simulink model "VoltageRegulator"  (R2018a)
settings: Solver=VariableStepAuto  StartTime=0.0  StopTime=10.0  RelTol=1e-3
libraries: elec_lib x6, pe_lib x4, fl_lib x3, nesl_utility x3
settings Model: Creator=Jayef  LastModifiedBy=Jayef

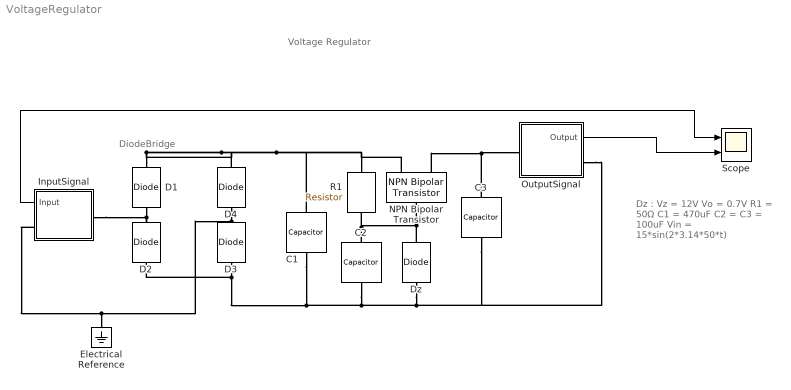
== system VoltageRegulator ==
  note: Voltage Regulator
  note: DiodeBridge
  note: Dz :
      | Vz = 12V
      | Vo = 0.7V
      |
      | R1 = 50Ω C1 = 470uF
      |
      | C2 = C3 = 100uF
      |
      | Vin = 15*sin(2*3.14*50*t)
  C1 : elec_lib/Passive Devices/Capacitor  enable_table=0  c=470 uF  Cvec=[1e-05, 1e-06] F  Vvec=[0, 10] V  CV_table_symmetry=1  C_tol=5  enable_C_tol=0  tol_distribution=1  nSigma=4  r=1e-6 Ohm  g=0 1/Ohm  enable_operating_limits=0  operating_limit_action=2  max_working_voltage_range=[-25, 25] V  power_rating=1 W  enable_faults=0  fault_action=1  Cscale_faulted=100  R_faulted=1e-3 Ohm  G_faulted=0 1/Ohm  tau_fault=1e-3 s  enable_temporal_fault=0  t_fault=1 s  enable_behavioral_fault=0  max_permissible_voltage_range=[-100, 100] V  t_fail_on_voltage=1 s  i_specify=off  i_priority=None  i=0 A  i_nominal_specify=off  i_nominal_unit=A  i_nominal_value=1  v_specify=off  v_priority=None  v=0 V  v_nominal_specify=off  v_nominal_unit=V  v_nominal_value=1  vc_specify=off  vc_priority=High  vc=0 V  vc_nominal_specify=off  vc_nominal_unit=V  vc_nominal_value=1
  C2 : elec_lib/Passive Devices/Capacitor  enable_table=0  c=100 uF  Cvec=[1e-05, 1e-06] F  Vvec=[0, 10] V  CV_table_symmetry=1  C_tol=5  enable_C_tol=0  tol_distribution=1  nSigma=4  r=1e-6 Ohm  g=0 1/Ohm  enable_operating_limits=0  operating_limit_action=2  max_working_voltage_range=[-25, 25] V  power_rating=1 W  enable_faults=0  fault_action=1  Cscale_faulted=100  R_faulted=1e-3 Ohm  G_faulted=0 1/Ohm  tau_fault=1e-3 s  enable_temporal_fault=0  t_fault=1 s  enable_behavioral_fault=0  max_permissible_voltage_range=[-100, 100] V  t_fail_on_voltage=1 s  i_specify=off  i_priority=None  i=0 A  i_nominal_specify=off  i_nominal_unit=A  i_nominal_value=1  v_specify=off  v_priority=None  v=0 V  v_nominal_specify=off  v_nominal_unit=V  v_nominal_value=1  vc_specify=off  vc_priority=High  vc=0 V  vc_nominal_specify=off  vc_nominal_unit=V  vc_nominal_value=1
  C3 : elec_lib/Passive Devices/Capacitor  enable_table=0  c=100 uF  Cvec=[1e-05, 1e-06] F  Vvec=[0, 10] V  CV_table_symmetry=1  C_tol=5  enable_C_tol=0  tol_distribution=1  nSigma=4  r=1e-6 Ohm  g=0 1/Ohm  enable_operating_limits=0  operating_limit_action=2  max_working_voltage_range=[-25, 25] V  power_rating=1 W  enable_faults=0  fault_action=1  Cscale_faulted=100  R_faulted=1e-3 Ohm  G_faulted=0 1/Ohm  tau_fault=1e-3 s  enable_temporal_fault=0  t_fault=1 s  enable_behavioral_fault=0  max_permissible_voltage_range=[-100, 100] V  t_fail_on_voltage=1 s  i_specify=off  i_priority=None  i=0 A  i_nominal_specify=off  i_nominal_unit=A  i_nominal_value=1  v_specify=off  v_priority=None  v=0 V  v_nominal_specify=off  v_nominal_unit=V  v_nominal_value=1  vc_specify=off  vc_priority=High  vc=0 V  vc_nominal_specify=off  vc_nominal_unit=V  vc_nominal_value=1
  D{1..4} (4 alike) : pe_lib/Semiconductors/Fundamental Components/Diode  Vf=0.7 V  Ron=0.3 Ohm  Goff=1e-5 1/Ohm  N_series=1  N_parallel=1  Vf_equiv=0.8 V  Ron_equiv=0.001 Ohm  Goff_equiv=1e-5 1/Ohm
      settings: SourceProductName=Simscape Power Systems  SourceProductBaseCode=PS
  Dz : elec_lib/Semiconductor Devices/Diode  ModelType=2  Vf=.7 V  Ron=0.3 Ohm  Goff=1e-8 S  Rz=0.3 Ohm  Vz=12 V  C_PWL=5 pF  prmExp=1  I12=[.0137, .545] A  V12=[.6, .7] V  I1=0.0137 A  V1=0.6 V  IS=1e-12 A  ec=1  RS=0.01 Ohm  Tmeas=25 degC  BV=inf V  C_param=1  CJ0=5 pF  VJ=1 V  Mgrad=0.5  Vvec=[.1, 10, 100] V  Cvec=[3.5, 1, .4] pF  FC=0.5  Q_param=1  Irrm=-7.15 A  iF=4 A  didt=-750 A/us  trr=115 ns  TT=50 ns  tau=100 ns  T_param=1  IS_T2=1.25e-7 A  I1_T2=0.245 A  V1_T2=0.5 V  Tmeas2=125 degC  EG_param=1  EG=1.11 eV  XTI_param=1  XTI=3  dBVdT=0 V/K  Tdevice=25 degC  i_capacitor_specify=off  i_capacitor_priority=High  i_capacitor=0 A  i_capacitor_nominal_specify=off  i_capacitor_nominal_unit=A  i_capacitor_nominal_value=1  v_capacitor_specify=off  v_capacitor_priority=None  v_capacitor=0 V  v_capacitor_nominal_specify=off  v_capacitor_nominal_unit=V  v_capacitor_nominal_value=1  Rth=[0, 10] K/W  thermal_mass_parameterization=1  thermal_mass=[0, 1] J/K  thermal_time_constant=[0, 10] s  thermal_mass_initial_temperatures=[25, 25] degC
      settings: SourceProductName=Simscape Electronics  SourceProductBaseCode=SN
  Electrical Reference : fl_lib/Electrical/Electrical Elements/Electrical Reference
  InputSignal : Subsystem
  NPN Bipolar Transistor : elec_lib/Semiconductor Devices/NPN Bipolar Transistor  parameterization=1  prmDatasheet=1  prmEquCoeff=1  BF=100  IS=1e-14 A  ec=1  VAF=200 V  hfe=100  hoe=5e-5 1/Ohm  Ic_h=1 mA  Vce_h=5 V  V1=0.55 V  I1=0.5 mA  BR=1  Tmeas=25 degC  RC=0.01 Ohm  RE=1e-4 Ohm  RB=1 Ohm  C_BC=5 pF  C_BE=5 pF  TF=0 us  TR=0 us  hfe_T2=125  XTB=0  V1_T2=0.45 V  I1_T2=0.5 mA  Tmeas2=125 degC  EG=1.11 eV  XTI=3  TdeviceDatasheet=25 degC  TdeviceEquCoeff=25 degC  Rth=[ 0 10 ] K/W  thermal_mass_parameterization=1  thermal_mass=[ 0 1 ] J/K  thermal_time_constant=[ 0 10 ] s  thermal_mass_initial_temperatures=[ 25 25 ] degC
      settings: SourceProductName=Simscape Electronics  SourceProductBaseCode=SN
  OutputSignal : Subsystem
  R1 : elec_lib/Passive Devices/Resistor  R=50 Ohm  R_tol=5  enable_R_tol=0  tol_distribution=1  nSigma=4  enable_operating_limits=0  operating_limit_action=2  max_working_voltage=100 V  power_rating=1 W  enable_faults=0  fault_action=1  R_faulted=inf Ohm  enable_temporal_fault=0  t_fault=1 s  enable_behavioral_fault=0  max_permissible_current=1 A  t_fail_on_current=1 s  noise_mode=0  sample_time=1e-3 s  repeatability=1  auto_seed=2904386122  user_seed=0  Tdevice=25 degC  alpha=3.93e-3 1/K  Tmeas=25 degC  thermal_mass=100 J/K  power_derating_T1=70 degC  power_derating_T2=155 degC  operating_temperature_range_vec=[-50, 150] degC  temperature_specify=off  temperature_priority=High  temperature=298.15 K  temperature_nominal_specify=off  temperature_nominal_unit=K  temperature_nominal_value=1
  Scope : Scope  NumInputPorts=2
  wires:
  InputSignal/1(Input) -> Scope/1
  OutputSignal/1(Output) -> Scope/2
  connections:
  D1/RConn1 -- D4/RConn1 -- NPN Bipolar Transistor/RConn1 -- R1/LConn1 -- C1/LConn1
  D3/LConn1 -- OutputSignal/RConn1 -- C3/RConn1 -- Dz/LConn1 -- C2/RConn1 -- C1/RConn1 -- D2/LConn1
  C2/LConn1 -- NPN Bipolar Transistor/LConn1 -- Dz/RConn1 -- R1/RConn1
  NPN Bipolar Transistor/RConn2 -- C3/LConn1 -- OutputSignal/LConn1
  InputSignal/RConn1 -- D4/LConn1 -- D3/RConn1 -- Electrical Reference/LConn1
  D1/LConn1 -- InputSignal/LConn1 -- D2/RConn1

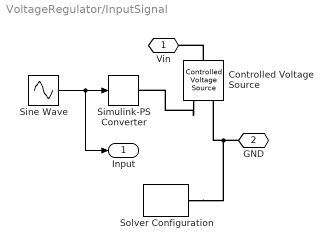
== system VoltageRegulator/InputSignal ==
  Controlled Voltage Source : fl_lib/Electrical/Electrical Sources/Controlled Voltage Source
  Simulink-PS Converter : nesl_utility/Simulink-PS Converter  PhysicalDomain=network_engine_domain  SubClassName=ps_input  LeftPortType=input  RightPortType=output  PseudoPeriodic=off  Frequencies=[]  NoiseDistribution=none  NoiseParameters=[]  Unit=1  AffineConversion=off  FilteringAndDerivatives=provide  SimscapeFilterOrder=1  InputFilterTimeConstant=0.001  UdotUserProvided=0
  Sine Wave : Sin  Amplitude=15  Frequency=2*3.14*50  SampleTime=0.00001
  Solver Configuration : nesl_utility/Solver Configuration  PhysicalDomain=network_engine_domain  SubClassName=solver  LeftPortType=input  RightPortType=generic  Tones=[]  Harmonics=[]  SimulateNoise=off  Profile=off  UseLocalSampling=off  EnableSwitchedLinearOptims=on  FrequencyDomain=off  UseCCode=off  RelTol=0.001  AbsTol=1e-06  MinStep=1e-09  ToWorkspace=off  RevertToSquareIcSolve=off  NumHomotopyIterations=100  PhasorMode=off  PhasorModeNumHarmonics=1  DoDC=off  ResidualTolerance=1e-09  UseLocalSolver=off  LocalSolverChoice=NE_BACKWARD_EULER_ADVANCER  LocalSolverSampleTime=0.001  DoFixedCost=off  MaxNonlinIter=3  MaxModeIter=2  LinearAlgebra=Sparse  EquationFormulation=NE_TIME_EF  DelaysMemoryBudget=1024  AutomaticFiltering=on  FilteringTimeConstant=0.001
  Vin : PMIOPort  Side=Left
  GND : PMIOPort  Port=2  Side=Right
  Input : Outport
  wires:
  Sine Wave/1 -> Input/1, Simulink-PS Converter/1
  connections:
  Controlled Voltage Source/RConn1 -- Simulink-PS Converter/RConn1
  GND/RConn1 -- Controlled Voltage Source/RConn2 -- Solver Configuration/RConn1
  Controlled Voltage Source/LConn1 -- Vin/RConn1

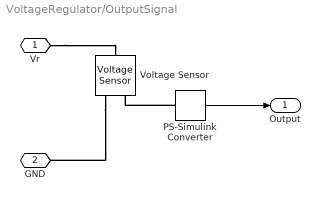
== system VoltageRegulator/OutputSignal ==
  PS-Simulink Converter : nesl_utility/PS-Simulink Converter  PhysicalDomain=network_engine_domain  SubClassName=ps_output  LeftPortType=input  RightPortType=output  PseudoPeriodic=off  Frequencies=[]  Unit=1  AffineConversion=off
  Voltage Sensor : fl_lib/Electrical/Electrical Sensors/Voltage Sensor
  Vr : PMIOPort  Side=Left
  GND : PMIOPort  Port=2  Side=Right
  Output : Outport
  wires:
  PS-Simulink Converter/1 -> Output/1
  connections:
  PS-Simulink Converter/LConn1 -- Voltage Sensor/RConn1
  Voltage Sensor/RConn2 -- GND/RConn1
  Vr/RConn1 -- Voltage Sensor/LConn1
